simulink model "stepFn1"  (R2024a)
settings: Solver=VariableStepAuto  StartTime=0.0  StopTime=10.0  RelTol=1e-3
settings Model: Creator=pouya  LastModifiedBy=pouya

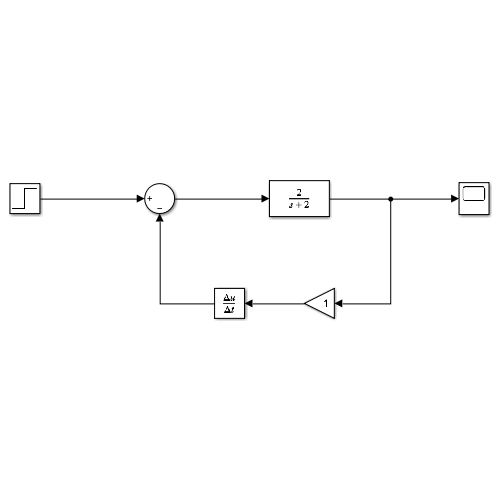
[thumbnail: Simulink's stored preview of the top-level diagram]
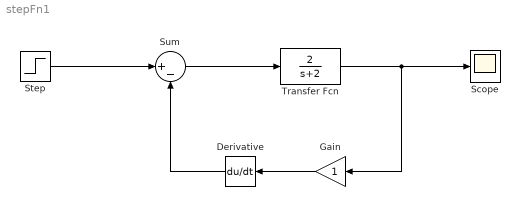
== system stepFn1 ==
  Derivative : Derivative
  Gain : Gain
  Scope : Scope
  Step : Step  Time=0  SampleTime=0
  Sum : Sum  Inputs=|+-
  Transfer Fcn : TransferFcn  Numerator=[2]  Denominator=[1 2]
  wires:
  Sum/1 -> Transfer Fcn/1
  Transfer Fcn/1 -> Scope/1, Gain/1
  Gain/1 -> Derivative/1
  Derivative/1 -> Sum/2
  Step/1 -> Sum/1
